simulink model "FinalProject"  (R2020a)
settings: Solver=FixedStepAuto  StartTime=0.0  StopTime=500  RelTol=1e-3
libraries: simulink_extras x2
settings Model: Creator=Richard  LastModifiedBy=Richard
settings DebuggingCC: AlgebraicLoopMsg=none

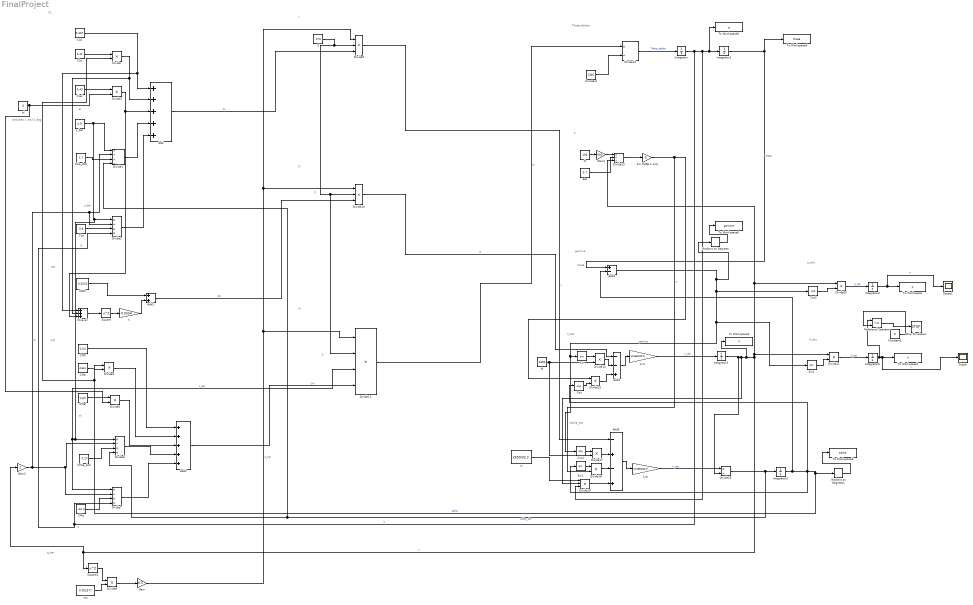
== system FinalProject ==
  note: h_dot
  note: p_dot
  note: alpha_dot
  note: V_dot
  note: theta
  note: between 1 and 2 deg
  note: T
  note: gamma
  note: Theta_dotdot
  note: S
  note: L
  note: q_bar
  note: el
  note: CM
  note: c_bar
  note: CD
  note: q
  note: el
  note: CL
  note: q
  note: D
  note: S
  note: M
  1/m : Gain  Gain=1/(2650/32.2)
  "1/m " : Gain  Gain=1/(2650/32.2)
  Add : Sum  Inputs=+++++
  Add1 : Sum
  Add2 : Sum  Inputs=+++++
  Add3 : Sum  Inputs=+-
  Add4 : Sum  Inputs=--+
  Add5 : Sum  Inputs=-+-+
  CDM : Constant  Value=0.0223
  CL(a,el) : Sum  Inputs=+++
  CL(a_dot) : Constant  Value=1.7
  CL0 : Constant  Value=0.307
  CLa : Constant  Value=4.41
  CLel : Constant  Value=0.43
  CLq : Constant  Value=3.9
  CM(a_dot) : Constant  Value=-7.27
  CM0 : Constant  Value=0.04
  CMa : Constant  Value=-0.613
  CMel : Constant  Value=-1.122
  CMq : Constant  Value=-12.4
  Constant : Constant  Value=1346
  Constant1 : Constant  Value=0
  Cos : Trigonometry  Operator=cos
  Cos1 : Trigonometry  Operator=cos
  Cos2 : Trigonometry  Operator=cos
  Divide{,3..5,8,14..15,17..18,20..21} (11 alike) : Product  Inputs=**
  Divide{1..2,6..7} (4 alike) : Product  Inputs=*/**
  Divide10 : Product  Inputs=***
  Divide11 : Product  Inputs=****
  Divide12 : Product  Inputs=*/
  Divide13 : Product  Inputs=**/
  Divide16 : Product  Inputs=*/
  Divide19 : Product  Inputs=***
  Divide9 : Product  Inputs=***
  For CASE 1 only : Gain  Gain=0
  Gain : Gain  Gain=0.5
  Gain1 : Gain  Gain=550
  Gain2 : Gain  Gain=2
  Integrator{,1,3..4} (4 alike) : Integrator
  Integrator2 : Integrator  InitialCondition=100*5280/3600
  Integrator5 : Integrator  InitialCondition=2000
  Radians to Degrees : simulink_extras/Transformations/Radians to Degrees
  Radians to Degrees1 : simulink_extras/Transformations/Radians to Degrees
  Relational Operator : RelationalOperator  Operator=<=  OutDataTypeStr=boolean  RndMeth=Simplest
  S : Constant  Value=174
  Scope : Scope
  Scope1 : Scope
  Sin : Trigonometry
  Sin1 : Trigonometry
  Sin2 : Trigonometry
  Square : Math  Operator=square  SaturateOnIntegerOverflow=on
  Square1 : Math  Operator=square  SaturateOnIntegerOverflow=on
  Stop Simulation : Stop
  To Workspace : ToWorkspace  VariableName=p  SampleTime=.01
      settings: Save2DSignal=2-D array (concatenate along first dimension)
  To Workspace1 : ToWorkspace  VariableName=h  SampleTime=.01
      settings: Save2DSignal=2-D array (concatenate along first dimension)
  To Workspace2 : ToWorkspace  VariableName=V  SampleTime=.01
      settings: Save2DSignal=2-D array (concatenate along first dimension)
  To Workspace3 : ToWorkspace  VariableName=alpha  SampleTime=.01
      settings: Save2DSignal=2-D array (concatenate along first dimension)
  To Workspace4 : ToWorkspace  VariableName=theta  SampleTime=.01
      settings: Save2DSignal=2-D array (concatenate along first dimension)
  To Workspace5 : ToWorkspace  VariableName=q  SampleTime=.01
      settings: Save2DSignal=2-D array (concatenate along first dimension)
  To Workspace6 : ToWorkspace  VariableName=gamma  SampleTime=.01
      settings: Save2DSignal=2-D array (concatenate along first dimension)
  W : Constant  Value=2650
  c_bar : Constant  Value=4.9
  el : Constant  Value=0
  eta : Constant  Value=0.7
  k : Gain  Gain=0.0554
  m : Constant  Value=2650/32.2
  rho : Constant  Value=0.002377
  th : Constant  Value=100
  wires:
  CL0/1 -> CL(a,el)/1, Add/1
  Divide/1 -> CL(a,el)/2, Add/2
  Divide3/1 -> Add/3, CL(a,el)/3
  Divide1/1 -> Add/4
  Divide2/1 -> Add/5
  Add/1 -> Divide9/3  "CL"
  CLa/1 -> Divide/1
  CLel/1 -> Divide3/1
  CL(a_dot)/1 -> Divide1/3
  CLq/1 -> Divide2/3
  CDM/1 -> Add1/1
  Add1/1 -> Divide10/3  "CD"
  CL(a,el)/1 -> Square/1
  CMa/1 -> Divide4/1
  Square/1 -> k/1
  k/1 -> Add1/2
  CMel/1 -> Divide5/1
  el/1 -> Divide5/2, Divide3/2
  CM(a_dot)/1 -> Divide6/3
  Gain2/1 -> Divide1/2, Divide2/2, Divide7/2, Divide6/2  "2V"
  CMq/1 -> Divide7/3
  c_bar/1 -> Divide1/1, Divide7/1, Divide11/3, Divide6/1, Divide2/1  "c_bar"
  CM0/1 -> Add2/1
  Divide4/1 -> Add2/2
  Divide5/1 -> Add2/3
  Divide6/1 -> Add2/4
  Divide7/1 -> Add2/5
  Add2/1 -> Divide11/4  "CM"
  Gain/1 -> Divide11/1, Divide9/1, Divide10/1  "q_bar"
  Square1/1 -> Divide8/1
  rho/1 -> Divide8/2
  Divide8/1 -> Gain/1
  S/1 -> Divide10/2, Divide11/2, Divide9/2
  Divide11/1 -> Divide12/1  "M"
  Divide9/1 -> Add5/1  "L"
  Divide10/1 -> Add4/1  "D"
  Constant/1 -> Divide12/2
  Divide12/1 -> Integrator/1  "Theta_dotdot"
  Integrator/1 -> Divide19/3, To Workspace5/1, Integrator1/1, Divide7/4, Divide2/4  "q"
  Integrator1/1 -> To Workspace4/1, Add3/1  "Theta"
  th/1 -> Gain1/1
  Gain1/1 -> Divide13/1
  eta/1 -> Divide13/2
  Divide13/1 -> For CASE 1 only/1
  For CASE 1 only/1 -> Divide18/2, Divide15/1  "T"
  Add3/1 -> Radians to Degrees/1, Cos2/1, Sin2/1, Cos1/1, Sin/1  "gamma"
  Add4/1 -> 1/m/1
  Sin/1 -> Divide14/1
  W/1 -> Divide14/2, Divide17/2
  Divide14/1 -> Add4/2
  Cos/1 -> Divide15/2
  Divide15/1 -> Add4/3
  1/m/1 -> Integrator2/1  "V_dot"
  Integrator2/1 -> Divide16/2, Divide19/2, To Workspace2/1, Divide20/1, Divide13/3, Divide21/1, Square1/1, Gain2/1  "V"
  Add5/1 -> "1/m "/1
  "1/m "/1 -> Divide16/1  "V_dot"
  Divide16/1 -> Divide1/4, Divide6/4, Integrator3/1  "alpha_dot"
  Integrator3/1 -> Add3/2, Radians to Degrees1/1, Divide/2, Divide4/2, Cos/1, Sin1/1  "alpha"
  Cos1/1 -> Divide17/1
  Divide17/1 -> Add5/2
  Sin1/1 -> Divide18/1
  Divide18/1 -> Add5/3
  m/1 -> Divide19/1
  Divide19/1 -> Add5/4
  Cos2/1 -> Divide20/2
  Divide20/1 -> Integrator4/1  "p_dot"
  Integrator4/1 -> Scope1/1, To Workspace/1  "p"
  Sin2/1 -> Divide21/2
  Divide21/1 -> Integrator5/1  "h_dot"
  Integrator5/1 -> To Workspace1/1, Scope/1, Relational Operator/1  "h"
  Constant1/1 -> Relational Operator/2
  Relational Operator/1 -> Stop Simulation/1
  Radians to Degrees/1 -> To Workspace6/1
  Radians to Degrees1/1 -> To Workspace3/1
